simulink model "ObservadorPlantaBuenazo_bienHecho"  (R2016a)
settings: Solver=ode45  StartTime=0.0  StopTime=10  MaxStep=0.01  RelTol=1e-3
values from neighbouring files (symbols this model uses):
  A = [0 1; -Mt/I -Kf/I]    [HinfPlantSeguroa.m]    (also in HinfPlanta.m)
  B = [0; L1/I]    [HinfPlantSeguroa.m]    (also in HinfPlanta.m)
  C = [1 0]    [HinfPlantSeguroa.m]    (also in HinfPlanta.m)
  L = G1*K1    [HinfPlantSeguroa.m]    (also in HinfPlanta.m)
settings Model: Creator=i95sa  LastModifiedBy=i95sa
settings DataIOCC: SaveFormat=StructureWithTime
settings DebuggingCC: FcnCallInpInsideContextMsg=EnableAllAsWarning
settings HardwareCC: ProdWordSize=32  ProdHWDeviceType=Specified
settings ConfigComp: CovSFcnEnable=off

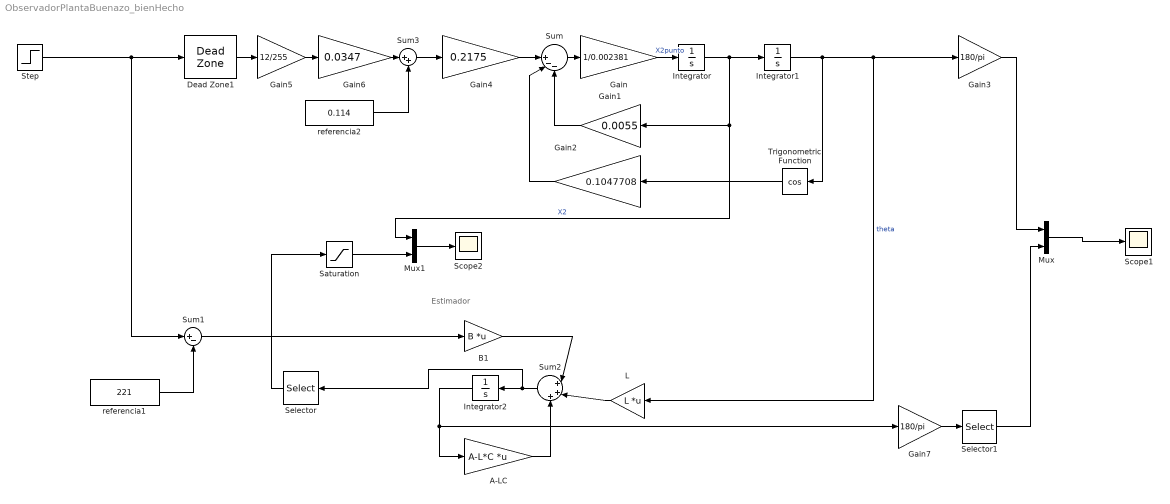
== system ObservadorPlantaBuenazo_bienHecho ==
  note: Estimador
  A-LC : Gain  Gain=A-L*C  Multiplication=Matrix(K*u)
  B1 : Gain  Gain=B  Multiplication=Matrix(K*u)
  Dead Zone1 : DeadZone  LowerValue=0  UpperValue=0  SaturateOnIntegerOverflow=on
  Gain : Gain  Gain=1/0.002381
  Gain1 : Gain  Gain=0.0055
  Gain2 : Gain  Gain=0.1047708
  Gain3 : Gain  Gain=180/pi
  Gain4 : Gain  Gain=0.2175
  Gain5 : Gain  Gain=12/255
  Gain6 : Gain  Gain=0.0347
  Gain7 : Gain  Gain=180/pi
  Integrator : Integrator
  Integrator1 : Integrator  InitialCondition=-0.65
  Integrator2 : Integrator
  L : Gain  Gain=L  Multiplication=Matrix(K*u)
  Mux : Mux  Inputs=2
  Mux1 : Mux  Inputs=2
  Saturation : Saturate  UpperLimit=inf  LowerLimit=-1
  Scope1 : Scope
  Scope2 : Scope
  Selector : Selector  InputPortWidth=2  IndexOptions=Index vector (dialog)  Indices=[1]  OutputSizes=1
  Selector1 : Selector  InputPortWidth=2  IndexOptions=Index vector (dialog)  Indices=[1]  OutputSizes=1
  Step : Step  Time=0  After=221  SampleTime=0
  Sum : Sum  Inputs=||+--
  Sum1 : Sum  Inputs=|+-
  Sum2 : Sum  Inputs=|+++
  Sum3 : Sum  Inputs=|++
  Trigonometric Function : Trigonometry  Operator=cos
  referencia1 : Constant  Value=221
  referencia2 : Constant  Value=0.114
  wires:
  Sum/1 -> Gain/1
  Gain/1 -> Integrator/1  "X2punto"
  Integrator/1 -> Mux1/1, Gain1/1, Integrator1/1  "X2"
  Trigonometric Function/1 -> Gain2/1
  Gain1/1 -> Sum/3
  Integrator1/1 -> L/1, Gain3/1, Trigonometric Function/1  "theta"
  Gain2/1 -> Sum/2
  Gain4/1 -> Sum/1
  referencia2/1 -> Sum3/2
  Sum3/1 -> Gain4/1
  Gain5/1 -> Gain6/1
  Gain6/1 -> Sum3/1
  Dead Zone1/1 -> Gain5/1
  Gain3/1 -> Mux/1
  Mux/1 -> Scope1/1
  Mux1/1 -> Scope2/1
  Step/1 -> Sum1/1, Dead Zone1/1
  B1/1 -> Sum2/1
  Integrator2/1 -> A-LC/1, Gain7/1
  A-LC/1 -> Sum2/3
  L/1 -> Sum2/2
  Gain7/1 -> Selector1/1
  Sum2/1 -> Selector/1, Integrator2/1
  Selector/1 -> Saturation/1
  Selector1/1 -> Mux/2
  referencia1/1 -> Sum1/2
  Sum1/1 -> B1/1
  Saturation/1 -> Mux1/2
